simulink model "Template_Matching"  (R2020a)
settings: Solver=VariableStepAuto  StartTime=0.0  StopTime=10  RelTol=1e-3
libraries: simulink x2, dspfdesign x1
settings Model: Creator=sbuccelli  LastModifiedBy=diflo

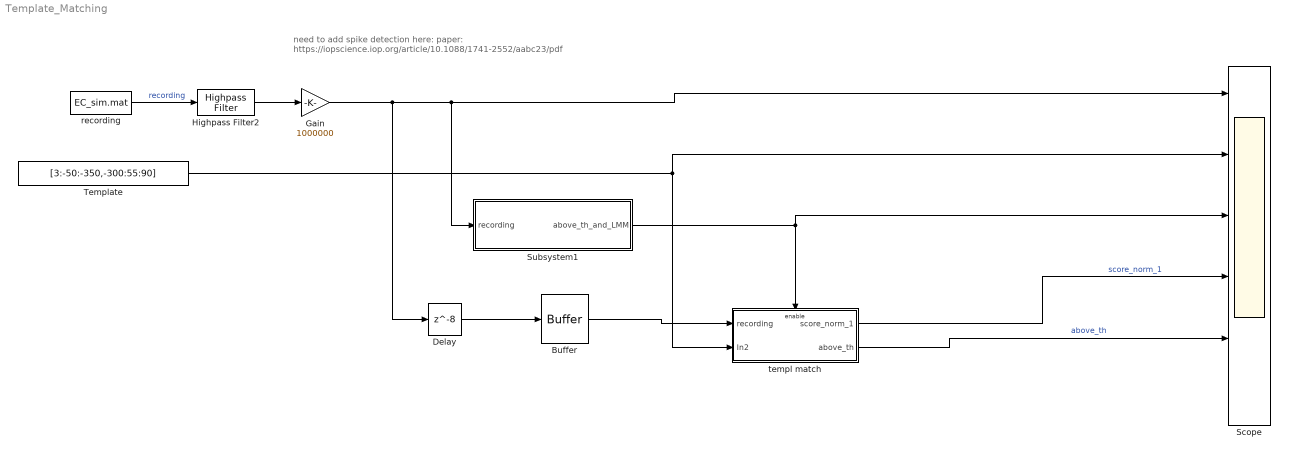
== system Template_Matching ==
  note: need to add spike detection here:
      | paper: https://iopscience.iop.org/article/10.1088/1741-2552/aabc23/pdf
  Buffer : Buffer  N=16  OutputFrames=off
  Delay : Delay  DelayLength=8  InitialCondition=0
  Gain : Gain  Gain=1000000
  Highpass Filter2 : dspfdesign/Highpass Filter  FilterType=IIR  DesignForMinimumOrder=off  FilterOrder=3  StopbandFrequency=1  PassbandFrequency=300  StopbandAttenuation=80  PassbandRipple=0.1  InheritSampleRate=off  SampleRate=30000  SimulateUsing=Interpreted execution  roundingMode=Floor  coeffsDataTypeStr=fixdt(1,16)
  Scope : Scope  NumInputPorts=6
  Subsystem1 : Subsystem
  Template : Constant  Value=[3:-50:-350,-300:55:90]  SampleTime=1/30000
  recording : FromFile  FileName=EC_sim.mat  SampleTime=1/30000
  templ match : Subsystem
  wires:
  Template/1 -> templ match/2(In2), Scope/2
  recording/1 -> Highpass Filter2/1  "recording"
  templ match/1(score_norm_1) -> Scope/4  "score_norm_1"
  templ match/2(above_th) -> Scope/5  "above_th"
  Subsystem1/1(above_th_and_LMM) -> templ match/Enable, Scope/3
  Highpass Filter2/1 -> Gain/1
  Gain/1 -> Scope/1, Subsystem1/1(recording), Delay/1
  ? -> Scope/6
  Delay/1 -> Buffer/1
  Buffer/1 -> templ match/1(recording)

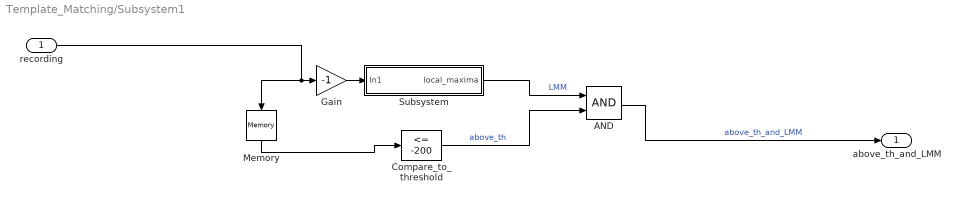
== system Template_Matching/Subsystem1 ==
  recording : Inport
  AND : Logic  AllPortsSameDT=off  OutDataTypeStr=boolean
  Compare_to_threshold : simulink/Logic and Bit Operations/Compare To Constant  relop=<=  const=-200  OutDataTypeStr=boolean
  Gain : Gain  Gain=-1
  Memory : Memory  InheritSampleTime=on
  Subsystem : Subsystem
  above_th_and_LMM : Outport
  wires:
  recording/1 -> Memory/1, Gain/1
  AND/1 -> above_th_and_LMM/1  "above_th_and_LMM"
  Subsystem/1(local_maxima) -> AND/1  "LMM"
  Gain/1 -> Subsystem/1(In1)
  Compare_to_threshold/1 -> AND/2  "above_th"
  Memory/1 -> Compare_to_threshold/1

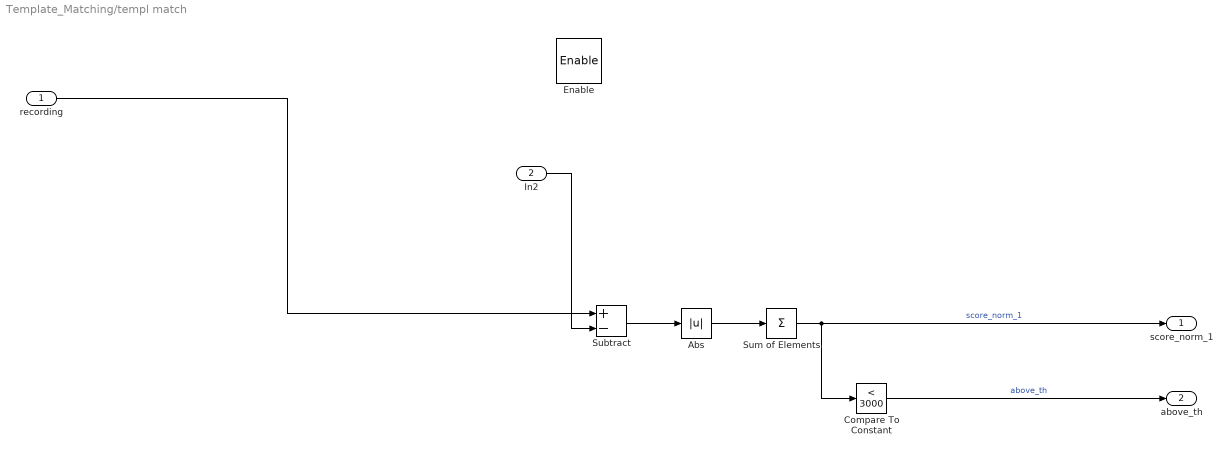
== system Template_Matching/templ match ==
  recording : Inport
  In2 : Inport  Port=2
  Enable : EnablePort  StatesWhenEnabling=reset
  Abs : Abs
  Compare To Constant : simulink/Logic and Bit Operations/Compare To Constant  relop=<  const=3000  OutDataTypeStr=boolean
  Subtract : Sum  Inputs=+-
  Sum of Elements : Sum  Inputs=+
  score_norm_1 : Outport  OutputWhenDisabled=reset  InitialOutput=0
  above_th : Outport  Port=2  OutputWhenDisabled=reset  InitialOutput=0
  wires:
  Compare To Constant/1 -> above_th/1  "above_th"
  Sum of Elements/1 -> score_norm_1/1, Compare To Constant/1  "score_norm_1"
  Subtract/1 -> Abs/1
  In2/1 -> Subtract/2
  Abs/1 -> Sum of Elements/1
  recording/1 -> Subtract/1

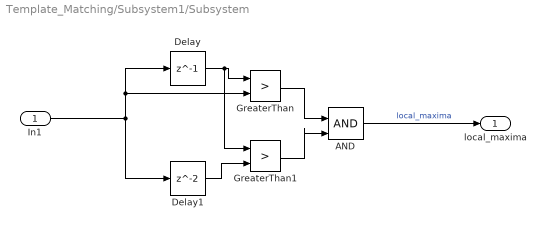
== system Template_Matching/Subsystem1/Subsystem ==
  In1 : Inport
  AND : Logic  IconShape=distinctive  AllPortsSameDT=off  OutDataTypeStr=boolean
  Delay : Delay  DelayLength=1
  Delay1 : Delay
  GreaterThan : RelationalOperator  Operator=>  OutDataTypeStr=boolean  RndMeth=Simplest
  GreaterThan1 : RelationalOperator  Operator=>  OutDataTypeStr=boolean  RndMeth=Simplest
  local_maxima : Outport
  wires:
  Delay1/1 -> GreaterThan1/2
  GreaterThan1/1 -> AND/2
  GreaterThan/1 -> AND/1
  Delay/1 -> GreaterThan1/1, GreaterThan/1
  AND/1 -> local_maxima/1  "local_maxima"
  In1/1 -> Delay/1, GreaterThan/2, Delay1/1
